simulink model "SimulinkBlockDiagram_ece3710_FINAL"  (R2022a)
settings: Solver=VariableStepAuto  StartTime=0.0  StopTime=130  FixedStep=1e-4  RelTol=1e-3
values from neighbouring files (symbols this model uses):
  B = 100e-6    (= 0.0001)    [DC_Motor_Parameters_FINAL.m]
  Gear = 7.5    [DC_Motor_Parameters_FINAL.m]
  J = 0.0026    [DC_Motor_Parameters_FINAL.m]
  Ke = 590e-6    (= 0.00059)    [DC_Motor_Parameters_FINAL.m]
  Ki = z*Kp    [DC_Motor_Parameters_FINAL.m]
  Kp = 0.00861    [DC_Motor_Parameters_FINAL.m]
  Kt = 590e-6    (= 0.00059)    [DC_Motor_Parameters_FINAL.m]
  La = 26e-6    (= 2.6e-05)    [DC_Motor_Parameters_FINAL.m]
  Ra = 0.008    [DC_Motor_Parameters_FINAL.m]
  SensorGain = 1    [DC_Motor_Parameters_FINAL.m]
settings Model: Creator=jkeus  LastModifiedBy=jkeus

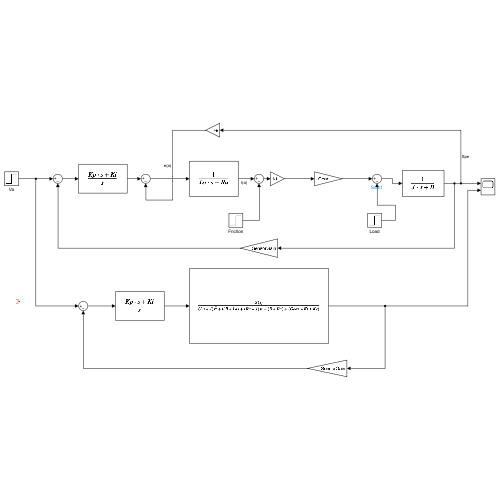
[thumbnail: Simulink's stored preview of the top-level diagram]
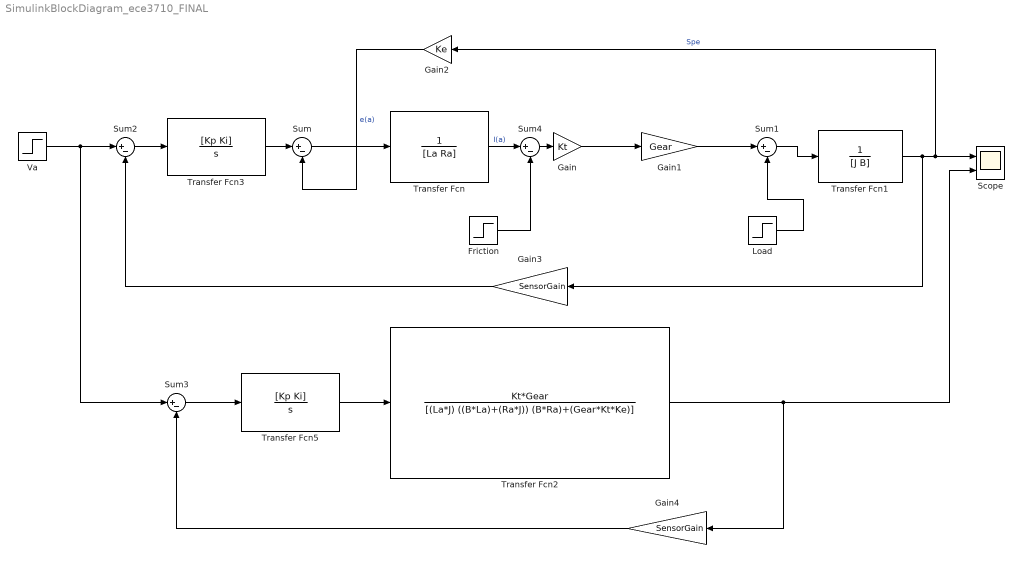
== system SimulinkBlockDiagram_ece3710_FINAL ==
  Friction : Step  After=0.01  SampleTime=0
  Gain : Gain  Gain=Kt
  Gain1 : Gain  Gain=Gear
  Gain2 : Gain  Gain=Ke
  Gain3 : Gain  Gain=SensorGain
  Gain4 : Gain  Gain=SensorGain
  Load : Step  Time=50  After=0.05  SampleTime=0
  Scope : Scope  NumInputPorts=2
  Sum{,1..4} (5 alike) : Sum  Inputs=|+-
  Transfer Fcn : TransferFcn  Denominator=[La Ra]
  Transfer Fcn1 : TransferFcn  Denominator=[J B]
  Transfer Fcn2 : TransferFcn  Numerator=Kt*Gear  Denominator=[(La*J) ((B*La)+(Ra*J)) (B*Ra)+(Gear*Kt*Ke)]
  Transfer Fcn3 : TransferFcn  Numerator=[Kp Ki]  Denominator=[1 0]
  Transfer Fcn5 : TransferFcn  Numerator=[Kp Ki]  Denominator=[1 0]
  Va : Step  Time=5  After=100  SampleTime=0
  wires:
  Sum/1 -> Transfer Fcn/1
  Transfer Fcn/1 -> Sum4/1  "I(a)"
  Gain/1 -> Gain1/1
  Load/1 -> Sum1/2
  Sum1/1 -> Transfer Fcn1/1
  Transfer Fcn1/1 -> Gain3/1, Scope/1, Gain2/1  "Spe"
  Gain2/1 -> Sum/2  "e(a)"
  Gain1/1 -> Sum1/1
  Gain4/1 -> Sum3/2
  ? -> ?
  Sum3/1 -> Transfer Fcn5/1
  Friction/1 -> Sum4/2
  Sum4/1 -> Gain/1
  Va/1 -> Sum3/1, Sum2/1
  Transfer Fcn2/1 -> Gain4/1, Scope/2
  Sum2/1 -> Transfer Fcn3/1
  Transfer Fcn3/1 -> Sum/1
  Gain3/1 -> Sum2/2
  Transfer Fcn5/1 -> Transfer Fcn2/1
